simulink model "SkywalkerX8_Longitudinal_Algebraic_Control"  (R2018a)
settings: Solver=FixedStepAuto  StartTime=0.0  StopTime=10.0  FixedStep=0.02  RelTol=1e-3
undefined symbols (not defined in the file): SkywalkerX8
libraries: simulink x3
settings Model: Creator=David  LastModifiedBy=David

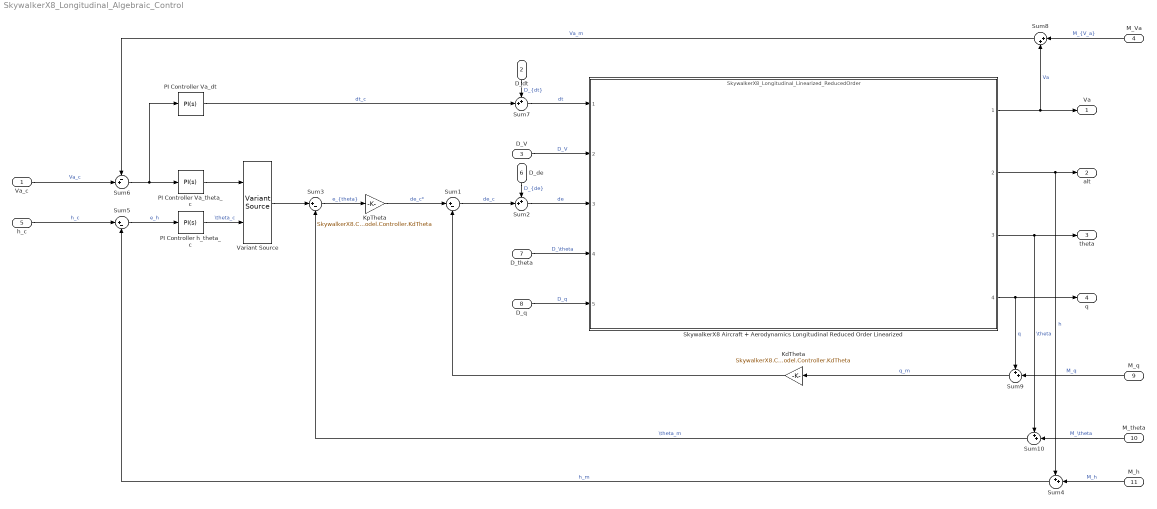
== system SkywalkerX8_Longitudinal_Algebraic_Control ==
  Va_c : Inport
  D_dt : Inport  Port=2
  D_V : Inport  Port=3
  M_Va : Inport  Port=4
  h_c : Inport  Port=5
  D_de : Inport  Port=6
  D_theta : Inport  Port=7
  D_q : Inport  Port=8
  M_q : Inport  Port=9
  M_theta : Inport  Port=10
  M_h : Inport  Port=11
  KdTheta : Gain  Gain=SkywalkerX8.Control.Longitudinal.AlgebraicDesign.ReducedOrderModel.Controller.KdTheta
  KpTheta : Gain  Gain=SkywalkerX8.Control.Longitudinal.AlgebraicDesign.ReducedOrderModel.Controller.KdTheta
  PI Controller Va_dt : simulink/Continuous/PID Controller  Controller=PI  TimeDomain=Continuous-time  SampleTime=-1  IntegratorMethod=Forward Euler  FilterMethod=Forward Euler  Form=Parallel  UseFilter=on  ControllerParametersSource=internal  P=SkywalkerX8.Control.Longitudinal.AlgebraicDesign.ReducedOrderModel.Controller.KpV  I=SkywalkerX8.Control.Longitudinal.AlgebraicDesign.ReducedOrderModel.Controller.KiV  D=0  N=100  InitialConditionSource=internal  InitialConditionForIntegrator=0  InitialConditionForFilter=0  ExternalReset=none  LimitOutput=off  UpperSaturationLimit=inf  LowerSaturationLimit=-inf  LinearizeAsGain=on  AntiWindupMode=none  Kb=1  TrackingMode=off  Kt=1  PParamMin=[]  PParamMax=[]  IParamMin=[]  IParamMax=[]  DParamMin=[]  DParamMax=[]  NParamMin=[]  NParamMax=[]  KbParamMin=[]  KbParamMax=[]  KtParamMin=[]  KtParamMax=[]  POutMin=[]  POutMax=[]  IOutMin=[]  IOutMax=[]  DOutMin=[]  DOutMax=[]  NOutMin=[]  NOutMax=[]  KbOutMin=[]  KbOutMax=[]  KtOutMin=[]  KtOutMax=[]  IntegratorOutMin=[]  IntegratorOutMax=[]  FilterOutMin=[]  FilterOutMax=[]  SumOutMin=[]  SumOutMax=[]  SumI1OutMin=[]  SumI1OutMax=[]  SumI2OutMin=[]  SumI2OutMax=[]  SumI3OutMin=[]  SumI3OutMax=[]  SumDOutMin=[]  SumDOutMax=[]  SaturationOutMin=[]  SaturationOutMax=[]  IntegratorContinuousStateAttributes=''  IntegratorStateMustResolveToSignalObject=off  IntegratorRTWStateStorageClass=Auto  FilterContinuousStateAttributes=''  FilterStateMustResolveToSignalObject=off  FilterRTWStateStorageClass=Auto  DifferentiatorICPrevScaledInput=0  DifferentiatorOutMin=[]  DifferentiatorOutMax=[]  FilterDiffOutCoefMin=[]  FilterDiffOutCoefMax=[]  SumDenOutMin=[]  SumDenOutMax=[]  SumNumOutMin=[]  SumNumOutMax=[]  ReciprocalOutMin=[]  ReciprocalOutMax=[]  DivideOutMin=[]  DivideOutMax=[]  TunerSelectOption=Transfer Function Based (PID Tuner App)
  PI Controller Va_theta_c : simulink/Continuous/PID Controller  Controller=PI  TimeDomain=Continuous-time  SampleTime=-1  IntegratorMethod=Forward Euler  FilterMethod=Forward Euler  Form=Parallel  UseFilter=on  ControllerParametersSource=internal  P=SkywalkerX8.Control.Longitudinal.AlgebraicDesign.ReducedOrderModel.Controller.KpV2  I=SkywalkerX8.Control.Longitudinal.AlgebraicDesign.ReducedOrderModel.Controller.KiV2  D=0  N=100  InitialConditionSource=internal  InitialConditionForIntegrator=0  InitialConditionForFilter=0  ExternalReset=none  LimitOutput=off  UpperSaturationLimit=inf  LowerSaturationLimit=-inf  LinearizeAsGain=on  AntiWindupMode=none  Kb=1  TrackingMode=off  Kt=1  PParamMin=[]  PParamMax=[]  IParamMin=[]  IParamMax=[]  DParamMin=[]  DParamMax=[]  NParamMin=[]  NParamMax=[]  KbParamMin=[]  KbParamMax=[]  KtParamMin=[]  KtParamMax=[]  POutMin=[]  POutMax=[]  IOutMin=[]  IOutMax=[]  DOutMin=[]  DOutMax=[]  NOutMin=[]  NOutMax=[]  KbOutMin=[]  KbOutMax=[]  KtOutMin=[]  KtOutMax=[]  IntegratorOutMin=[]  IntegratorOutMax=[]  FilterOutMin=[]  FilterOutMax=[]  SumOutMin=[]  SumOutMax=[]  SumI1OutMin=[]  SumI1OutMax=[]  SumI2OutMin=[]  SumI2OutMax=[]  SumI3OutMin=[]  SumI3OutMax=[]  SumDOutMin=[]  SumDOutMax=[]  SaturationOutMin=[]  SaturationOutMax=[]  IntegratorContinuousStateAttributes=''  IntegratorStateMustResolveToSignalObject=off  IntegratorRTWStateStorageClass=Auto  FilterContinuousStateAttributes=''  FilterStateMustResolveToSignalObject=off  FilterRTWStateStorageClass=Auto  DifferentiatorICPrevScaledInput=0  DifferentiatorOutMin=[]  DifferentiatorOutMax=[]  FilterDiffOutCoefMin=[]  FilterDiffOutCoefMax=[]  SumDenOutMin=[]  SumDenOutMax=[]  SumNumOutMin=[]  SumNumOutMax=[]  ReciprocalOutMin=[]  ReciprocalOutMax=[]  DivideOutMin=[]  DivideOutMax=[]  TunerSelectOption=Transfer Function Based (PID Tuner App)
  PI Controller h_theta_c : simulink/Continuous/PID Controller  Controller=PI  TimeDomain=Continuous-time  SampleTime=-1  IntegratorMethod=Forward Euler  FilterMethod=Forward Euler  Form=Parallel  UseFilter=on  ControllerParametersSource=internal  P=SkywalkerX8.Control.Longitudinal.AlgebraicDesign.ReducedOrderModel.Controller.KpAlt  I=SkywalkerX8.Control.Longitudinal.AlgebraicDesign.ReducedOrderModel.Controller.KiAlt  D=0  N=100  InitialConditionSource=internal  InitialConditionForIntegrator=0  InitialConditionForFilter=0  ExternalReset=none  LimitOutput=off  UpperSaturationLimit=inf  LowerSaturationLimit=-inf  LinearizeAsGain=on  AntiWindupMode=none  Kb=1  TrackingMode=off  Kt=1  PParamMin=[]  PParamMax=[]  IParamMin=[]  IParamMax=[]  DParamMin=[]  DParamMax=[]  NParamMin=[]  NParamMax=[]  KbParamMin=[]  KbParamMax=[]  KtParamMin=[]  KtParamMax=[]  POutMin=[]  POutMax=[]  IOutMin=[]  IOutMax=[]  DOutMin=[]  DOutMax=[]  NOutMin=[]  NOutMax=[]  KbOutMin=[]  KbOutMax=[]  KtOutMin=[]  KtOutMax=[]  IntegratorOutMin=[]  IntegratorOutMax=[]  FilterOutMin=[]  FilterOutMax=[]  SumOutMin=[]  SumOutMax=[]  SumI1OutMin=[]  SumI1OutMax=[]  SumI2OutMin=[]  SumI2OutMax=[]  SumI3OutMin=[]  SumI3OutMax=[]  SumDOutMin=[]  SumDOutMax=[]  SaturationOutMin=[]  SaturationOutMax=[]  IntegratorContinuousStateAttributes=''  IntegratorStateMustResolveToSignalObject=off  IntegratorRTWStateStorageClass=Auto  FilterContinuousStateAttributes=''  FilterStateMustResolveToSignalObject=off  FilterRTWStateStorageClass=Auto  DifferentiatorICPrevScaledInput=0  DifferentiatorOutMin=[]  DifferentiatorOutMax=[]  FilterDiffOutCoefMin=[]  FilterDiffOutCoefMax=[]  SumDenOutMin=[]  SumDenOutMax=[]  SumNumOutMin=[]  SumNumOutMax=[]  ReciprocalOutMin=[]  ReciprocalOutMax=[]  DivideOutMin=[]  DivideOutMax=[]  TunerSelectOption=Transfer Function Based (PID Tuner App)
  SkywalkerX8 Aircraft + Aerodynamics Longitudinal Reduced Order Linearized : ModelReference  ModelNameDialog=SkywalkerX8_Longitudinal_Linearized_ReducedOrder  ModelReferenceVersion=1.72
      mask Display:
      | image('x8SkySunset.png', 'center')
      | 
      | port_label('input', 1, '\delta_t (Unitless)', 'texmode', 'on')
      | port_label('input', 2, 'D_V (m/s)', 'texmode', 'on')
      | port_label('input', 3, '\delta_e (rad)', 'texmode', 'on')
      | port_label('input', 4, 'D_\theta (rad)', 'texmode', 'on')
      | port_label('input', 5, 'D_q (rad/s)', 'texmode', 'on')
      | 
      | 
      | port_label('output', 1, 'V_a (m/s)', 'texmode', 'on')
      | port_label('output', 2, 'Altitude (m)', 'texmode', 'on')
      | port_label('output', 3, '\theta (rad)', 'texmode', 'on')
      | port_label('output', 4, 'q (rad/s)', 'texmode', 'on')
  Sum1 : Sum  Inputs=|+-
  Sum{2,4,7,9..10} (5 alike) : Sum  Inputs=++|
  Sum3 : Sum  Inputs=|+-
  Sum5 : Sum  Inputs=|+-
  Sum6 : Sum  Inputs=-+|
  Sum8 : Sum  Inputs=|++
  Variant Source : VariantSource
  Va : Outport
  alt : Outport  Port=2
  theta : Outport  Port=3
  q : Outport  Port=4
  wires:
  SkywalkerX8 Aircraft + Aerodynamics Longitudinal Reduced Order Linearized/3 -> theta/1, Sum10/1  "\\theta"
  SkywalkerX8 Aircraft + Aerodynamics Longitudinal Reduced Order Linearized/1 -> Sum8/2, Va/1  "Va"
  SkywalkerX8 Aircraft + Aerodynamics Longitudinal Reduced Order Linearized/2 -> Sum4/1, alt/1  "h"
  SkywalkerX8 Aircraft + Aerodynamics Longitudinal Reduced Order Linearized/4 -> q/1, Sum9/1  "q"
  KdTheta/1 -> Sum1/2
  D_theta/1 -> SkywalkerX8 Aircraft + Aerodynamics Longitudinal Reduced Order Linearized/4  "D_\\theta"
  Sum1/1 -> Sum2/2  "de_c"
  Sum2/1 -> SkywalkerX8 Aircraft + Aerodynamics Longitudinal Reduced Order Linearized/3  "de"
  D_de/1 -> Sum2/1  "D_{de}"
  KpTheta/1 -> Sum1/1  "de_c*"
  Sum3/1 -> KpTheta/1  "e_{theta}"
  Variant Source/1 -> Sum3/1
  M_h/1 -> Sum4/2  "M_h"
  Sum4/1 -> Sum5/2  "h_m"
  Sum5/1 -> PI Controller h_theta_c/1  "e_h"
  h_c/1 -> Sum5/1  "h_c"
  Va_c/1 -> Sum6/2  "Va_c"
  PI Controller h_theta_c/1 -> Variant Source/2  "\\theta_c"
  Sum6/1 -> PI Controller Va_dt/1, PI Controller Va_theta_c/1
  PI Controller Va_dt/1 -> Sum7/2  "dt_c"
  PI Controller Va_theta_c/1 -> Variant Source/1
  D_dt/1 -> Sum7/1  "D_{dt}"
  Sum7/1 -> SkywalkerX8 Aircraft + Aerodynamics Longitudinal Reduced Order Linearized/1  "dt"
  Sum8/1 -> Sum6/1  "Va_m"
  M_Va/1 -> Sum8/1  "M_{V_a}"
  M_q/1 -> Sum9/2  "M_q"
  D_q/1 -> SkywalkerX8 Aircraft + Aerodynamics Longitudinal Reduced Order Linearized/5  "D_q"
  Sum10/1 -> Sum3/2  "\\theta_m"
  M_theta/1 -> Sum10/2  "M_\\theta"
  D_V/1 -> SkywalkerX8 Aircraft + Aerodynamics Longitudinal Reduced Order Linearized/2  "D_V"
  Sum9/1 -> KdTheta/1  "q_m"
